simulink model "Predefined_with_GroundTruth_mod1acc"  (R2021b)
settings: Solver=VariableStepAuto  StartTime=0.0  StopTime=inf  RelTol=1e-3
model workspace (MAT data in the model file):
  firstWarning = 1
  originalScenarioChecksum = '114339432DE22364D47BB28FC96DC10C'
undefined symbols (not defined in the file or in its folder): Acceleration, ActorID, AngularVelocity, curvature, curvatureAhd, DefaultGear, DEND_B, DEND_S, DEND_T, direction, driving, gradbp, LF, LR, matlabshared, MAX_BRAKE, MAX_STEER, MAX_TORQUE, MCAR, MIN_BRAKE, MIN_STEER, MIN_TORQUE, NUMD_B, NUMD_S, NUMD_T, Pitch, Position, psi_o, R, Roll, RRdamp, scenario, SceneInfo, sigbuilder_block, STEER_RATIO, stopSign_ID, Tdead, thetaRefs, TL_ID, TrackWidth, Ts, ts, Vdead, Velocity, X_o, xRef2s, Y_o, Yaw, yRef2s
libraries: mpcsigdimcheck_private x10, drivingscenarioandsensors x8, drivingvehiclecontroller x2, slpidlib x2, simulink x2, trackingutilitieslib x2, mpclib x1, simulink_extras x1, drivinglib x1, autolibshared x1, vehdynlibviscommon x1, vehdynlibsteering x1
(part 3 of 3)

== stateflow chart Predefined_with_GroundTruth_mod1acc/Chart ==
  settings: updateMethod=DISCRETE  sampleTime=Ts
  state Stationary
    en:
    VelCmd = 0;
    CurrentVelCmd = VelCmd;
    Navi = 0;
  state Navigation
    state RailCrossing
      state Approaching
        en:
        %VelCmd = ApproachingSpeed;
        %CurrentVelCmd = VelCmd;
      state Stop
        en:
        VelCmd = 0;
        CurrentVelCmd = VelCmd;
        % apply brakes directly?
      state ExitScene
        en:
        ExitFlag = 1;
      state Transition
        en:
        VelCmd = SceneSpeed;
        CurrentVelCmd = VelCmd;
      (default) -> Navigation.RailCrossing.Approaching
      Navigation.RailCrossing.Approaching -> Navigation.RailCrossing.Stop : [D2S <= SDist]
      Navigation.RailCrossing.Stop -> Navigation.RailCrossing.Transition : [RRCross == 0]
      Navigation.RailCrossing.Transition -> Navigation.RailCrossing.ExitScene : [SDir == 'S']
    state RoundAbout
      state Approaching
        en:
        VelCmd = ApproachingSpeed;
        CurrentVelCmd = VelCmd;
      state Stop
        en:
        VelCmd = 0;
        CurrentVelCmd = VelCmd;
        % apply brakes directly?
      state ExitScene
        en:
        ExitFlag = 1;
      state Transition
        en:
        VelCmd = SceneSpeed;
        CurrentVelCmd = VelCmd;
      (default) -> Navigation.RoundAbout.Approaching
      Navigation.RoundAbout.Approaching -> Navigation.RoundAbout.Stop : [D2S <= SDist]
      Navigation.RoundAbout.Stop -> Navigation.RoundAbout.Transition : [Clear2Go == 1]
      Navigation.RoundAbout.Transition -> Navigation.RoundAbout.ExitScene : [SDir == 'S']
    state DestCheck
      en,du:
      % dest reached?
      (default) -> (junction 47)
      (junction 47) -> (junction 48) [order 1] : [D2D < 1]
      (junction 47) -> (junction 49) [order 2] : {DestReached = 0;}
      (junction 48) -> (junction 50) : {DestReached = 1;}
      (junction 50) -> (junction 49)
      (junction 49) -> (junction 51)
    state TrafficLight
      state Approaching
        en:
        VelCmd = ApproachingSpeed;
        CurrentVelCmd = VelCmd;
        % ACC to approach?
      state Stop
        en:
        VelCmd = 0;
        CurrentVelCmd = VelCmd;
        % apply brakes directly?
      state ExitScene
        en:
        ExitFlag = 1;
      state Transition
        en:
        VelCmd = SceneSpeed;
        CurrentVelCmd = VelCmd;
      (default) -> Navigation.TrafficLight.Approaching
      Navigation.TrafficLight.Approaching -> Navigation.TrafficLight.Stop : [D2S <= SDist]
      Navigation.TrafficLight.Stop -> Navigation.TrafficLight.Transition : [TLstate(4) == 3]
      Navigation.TrafficLight.Transition -> Navigation.TrafficLight.Stop [order 2] : [TLstate(4) == 1]
      Navigation.TrafficLight.Transition -> Navigation.TrafficLight.ExitScene [order 1] : [SDir == 'S']
    state SceneRecognition
      en :
      VelCmd = RoadSpeed;
      CurrentVelCmd = VelCmd;
      ExitFlag = 0;
    state Go
      en:
      VelCmd = RoadSpeed/2;
      CurrentVelCmd = VelCmd;
      % what if the destination is right after the scene?
    state StopSign
      state Approaching
        en:
        VelCmd = ApproachingSpeed;
        CurrentVelCmd = VelCmd;
      state Stop
        en:
        VelCmd = 0;
        CurrentVelCmd = VelCmd;
        % apply brakes directly?
      state ExitScene
        en:
        ExitFlag = 1;
      state Transition
        en:
        VelCmd = SceneSpeed;
        CurrentVelCmd = VelCmd;
      (default) -> Navigation.StopSign.Approaching
      Navigation.StopSign.Approaching -> Navigation.StopSign.Stop : [D2S <= 15]
      Navigation.StopSign.Stop -> Navigation.StopSign.Transition : [after(3,sec) && Clear2Go == 1]
      Navigation.StopSign.Transition -> Navigation.StopSign.ExitScene : [SDir == 'S']
    SceneRecognition -> RailCrossing [order 1] : [Scene == 3]
    RailCrossing -> Go : [ExitFlag == 1]
    SceneRecognition -> RoundAbout [order 2] : [Scene == 4]
    RoundAbout -> Go : [ExitFlag == 1]
    (default) -> DestCheck
    SceneRecognition -> TrafficLight [order 4] : [Scene == 1]
    DestCheck -> SceneRecognition : [DestReached == 0]
    SceneRecognition -> StopSign [order 3] : [Scene == 2]
    TrafficLight -> Go : [ExitFlag == 1]
    StopSign -> Go : [ExitFlag == 1]
    Go -> DestCheck : [Scene == 0]
  (default) -> Stationary
  Stationary -> Navigation : [Navigate == 1]
  Navigation -> Stationary : [Navigate == 0 || DestReached == 1]
  data: TLstate input; SDir input; ApproachingSpeed input; SceneSpeed input; SDist input; RRCross input; D2S input; Scene input; DestReached local; Navigate input; ExitFlag local; D2D input; Clear2Go input; RoadSpeed input; CurrentVelCmd local; Navi local; VelCmd output
